simulink model "sm_motor_grader_LiftAssembly"  (R2026a)
settings: Solver=daessc  StopTime=stopTime  AbsTol=1e-3  EnableMultiTasking=on
PostLoadFcn:
  | set_param([bdroot '/Inputs'],'test_source','Data')
  | set_param([bdroot '/Blade'],'popup_actuator_model','Position');
  | set_param([bdroot '/Drawbar'],'popup_actuator_model','Position');
  | set_param([bdroot '/LiftAssembly'],'popup_actuator_model','Position');
  | set_param([bdroot '/Actuation'],'popup_actuator_model','Position');
  | 
  | set_param([bdroot '/Actuation'],'popup_actuator_model_lift','Position');
  | set_param([bdroot '/LiftAssembly'],'popup_actuator_model_lift','Position');
  | 
  | set_param([bdroot '/Blade'],'popup_blade_ground_contact','None')
  | [activeTestCmds,motGradParams,stopTime] = sm_motor_grader_define_test(motGradParams,'GradingTest');
  | set_param(bdroot,'EnablePacing','off')
InitFcn:
  | sm_motor_grader_config_initLinkBarHole([bdroot '/LiftAssembly'],motGradParams)
undefined symbols (not defined in the file): motGradParams, X, Y, Z
libraries: sm_motor_grader_lib x23, sm_lib x5, nesl_utility x1, sm_vehicle_utilities_lib x1
Description:
  | Copyright 2025-2026 The MathWorks, Inc.
settings Model: Creator=smiller  LastModifiedBy=smiller
settings DataIOCC: SignalLoggingName=logsout_sm_motor_grader_LiftAssembly
settings DebuggingCC: SubsystemReferenceDiagnosticForUnitTest=warning
settings SimscapeCC: SimscapeNominalValues="[{\"value\":\"1\",\"unit\":\"A\"},{\"value\":\"1\",\"unit\":\"bar\"},{\"value\":\"1\",\"unit\":\"cm^2\"},{\"value\":\"1\",\"unit\":\"cm^3/s\"},{\"value\":\"1\",\"unit\":\"kJ/kg\"},{\"value\":\"1\",\"unit\":\"kW\"},{\"value\":\"1\",\"unit\":\"l\"},{\"value\":\"1\",\"unit\":\"N\"},{\"value\":\"1\",\"unit\":\"N*m\"},{\"value\":\"1\",\"unit\":\"V\"}]"  SimscapeLogSimulationStatistics=on  SimscapeLogName=simlog_sm_motor_grader_LiftAssembly
settings DiagnosticsConfigSet: SimMechanicsConflictingReferenceFrames=none
settings ExplorerConfigSet: InternalSimMechanicsExplorerSettings="<ExplorerConfiguration><canonicalview>default</canonicalview><AnimationSetting><BasePlaybackSpeed>1.0</BasePlaybackSpeed><PlaybackSpeedFactor>2.0</PlaybackSpeedFactor></AnimationSetting><TilePanel><TileInfo><Tiles Columns=\"2\" Count=\"3\" Rows=\"2\"><Column Weight=\"0.4582\"/><Column Weight=\"0.5418\"/><Row Weight=\"0.5\"/><Row Weight=\"0.5\"/><Tile Height=\"1\" Width=\"1\" X=\"0\" Y=\"0\"/><Tile Height=\"1\" Width=\"1\" X=\"0\" Y=\"1\"/><Tile Height=\"2\" Width=\"1\" X=\"1\" Y=\"0\"/></Tiles></TileInfo><SceneInfo><SceneViewer><BGColor><R>1</R><G>1</G><B>1</B></BGColor><Camera><DoPerspective>off</DoPerspective><Position><X>3.15625000000000044</X><Y>-5.23852944873328152e-32</Y><Z>5.47808148799324002</Z></Position><Center><X>3.15625000000000044</X><Y>-5.23852944873328152e-32</Y><Z>1.95604989013671826</Z></Center><Up><X>0</X><Y>1</Y><Z>0</Z></Up><ViewLimDist>1</ViewLimDist><YLim>2.57500000000000018</YLim><XLim>5.23247330960854118</XLim></Camera></SceneViewer><SceneViewer><BGColor><R>1</R><G>1</G><B>1</B></BGColor><Camera><DoPerspective>off</DoPerspective><Position><X>5.88186405066405449</X><Y>-3.15203884044619187</Y><Z>2.76526245490202038</Z></Position><Center><X>2.73782296717336138</X><Y>0.286756094621752888</Y><Z>1.70087354642860866</Z></Center><Up><X>-0.15027157805512012</X><Y>0.164359538497787616</Y><Z>0.974886862632591944</Z></Up><ViewLimDist>1</ViewLimDist><YLim>2.68459397792816157</YLim><XLim>5.45517139287181596</XLim></Camera></SceneViewer><SceneViewer><BGColor><R>1</R><G>1</G><B>1</B></BGColor><Camera><DoPerspective>off</DoPerspective><Position><X>-0.999784568848335997</X><Y>-2.06162958506149385</Y><Z>2.58851070440858155</Z></Position><Center><X>3.20360113123811852</X><Y>0.528944126100773016</Y><Z>1.25033386358515286</Z></Center><Up><X>0.230558082822453991</X><Y>0.124417230540786017</Y><Z>0.965071667385275167</Z></Up><ViewLimDist>1</ViewLimDist><YLim>3.04628555505233445</YLim><XLim>3.60646065711975128</XLim></Camera></SceneViewer></SceneInfo></TilePanel><MechEditorPanel><Cameras><Camera><Id>Camera1</Id><Value><Name>Track FixO FR</Name><NativeCamera><PositionTrackingFeature>Motor_Grader.Vehicle.Camera_Frames.Frame_FixO_FR.R</PositionTrackingFeature><CenterTrackingFeature>Motor_Grader.Vehicle.Camera_Frames.Frame_FixO_FR.R</CenterTrackingFeature><UpVectorTrackingFeature>Motor_Grader.Vehicle.Camera_Frames.Frame_FixO_FR.R</UpVectorTrackingFeature><CenterTrackingOrigin>off</CenterTrackingOrigin><CenterTrackingDirection>+X</CenterTrackingDirection><UpVectorTrackingDirection>+Z</UpVectorTrackingDirection></NativeCamera></Value></Camera><Camera><Id>Camera2</Id><Value><Name>Track FixO Right</Name><NativeCamera><PositionTrackingFeature>Motor_Grader.Vehicle.Camera_Frames.Frame_FixO_Right.R</PositionTrackingFeature><CenterTrackingFeature>Motor_Grader.Vehicle.Camera_Frames.Frame_FixO_Right.R</CenterTrackingFeature><UpVectorTrackingFeature>Motor_Grader.Vehicle.Camera_Frames.Frame_FixO_Right.R</UpVectorTrackingFeature><CenterTrackingOrigin>off</CenterTrackingOrigin><CenterTrackingDirection>+X</CenterTrackingDirection><UpVectorTrackingDirection>+Z</UpVectorTrackingDirection></NativeCamera></Value></Camera><Camera><Id>Camera3</Id><Value><Name>Track FixO RR</Name><NativeCamera><PositionTrackingFeature>Motor_Grader.Vehicle.Camera_Frames.Frame_FixO_RR.R</PositionTrackingFeature><CenterTrackingFeature>Motor_Grader.Vehicle.Camera_Frames.Frame_FixO_RR.R</CenterTrackingFeature><UpVectorTrackingFeature>Motor_Grader.Vehicle.Camera_Frames.Frame_FixO_RR.R</UpVectorTrackingFeature><CenterTrackingOrigin>off</CenterTrackingOrigin><CenterTrackingDirection>+X</CenterTrackingDirection><UpVectorTrackingDirection>+Z</UpVectorTrackingDirection></NativeCamera></Value></Camera><Camera><Id>Camera4</Id><Value><Name>Track FixO RL</Name><NativeCamera><PositionTrackingFeature>Motor_Grader.Vehicle.Camera_Frames.Frame_FixO_RL.R</PositionTrackingFeature><CenterTrackingFeature>Motor_Grader.Vehicle.Camera_Frames.Frame_FixO_RL.R</CenterTrackingFeature><UpVectorTrackingFeature>Motor_Grader.Vehicle.Camera_Frames.Frame_FixO_RL.R</UpVectorTrackingFeature><CenterTrackingOrigin>off</CenterTrackingOrigin><CenterTrackingDirection>+X</CenterTrackingDirection><UpVectorTrackingDirection>+Z</UpVectorTrackingDirection></NativeCamera></Value></Camera><Camera><Id>Camera5</Id><Value><Name>Track FixO Left</Name><NativeCamera><PositionTrackingFeature>Motor_Grader.Vehicle.Camera_Frames.Frame_FixO_Left.R</PositionTrackingFeature><CenterTrackingFeature>Motor_Grader.Vehicle.Camera_Frames.Frame_FixO_Left.R</CenterTrackingFeature><UpVectorTrackingFeature>Motor_Grader.Vehicle.Camera_Frames.Frame_FixO_Left.R</UpVectorTrackingFeature><CenterTrackingOrigin>off</CenterTrackingOrigin><CenterTrackingDirection>+X</CenterTrackingDirection><UpVectorTrackingDirection>+Z</UpVectorTrackingDirection></NativeCamera></Value></Camera><Camera><Id>Camera6</Id><Value><Name>Track FixO FL</Name><NativeCamera><PositionTrackingFeature>Motor_Grader.Vehicle.Camera_Frames.Frame_FixO_FL.R</PositionTrackingFeature><CenterTrackingFeature>Motor_Grader.Vehicle.Camera_Frames.Frame_FixO_FL.R</CenterTrackingFeature><UpVectorTrackingFeature>Motor_Grader.Vehicle.Camera_Frames.Frame_FixO_FL.R</UpVectorTrackingFeature><CenterTrackingOrigin>off</CenterTrackingOrigin><CenterTrackingDirection>+X</CenterTrackingDirection><UpVectorTrackingDirection>+Z</UpVectorTrackingDirection></NativeCamera></Value></Camera><Camera><Id>Camera7</Id><Value><Name>Track FixO Top</Name><NativeCamera><PositionTrackingFeature>Motor_Grader.Vehicle.Camera_Frames.Frame_FixO_Top.R</PositionTrackingFeature><CenterTrackingFeature>Motor_Grader.Vehicle.Camera_Frames.Frame_FixO_Top.R</CenterTrackingFeature><UpVectorTrackingFeature>Motor_Grader.Vehicle.Camera_Frames.Frame_FixO_Top.R</UpVectorTrackingFeature><CenterTrackingOrigin>off</CenterTrackingOrigin><CenterTrackingDirection>+X</CenterTrackingDirection><UpVectorTrackingDirection>+Z</UpVectorTrackingDirection></NativeCamera></Value></Camera><Camera><Id>Camera8</Id><Value><Name>Track FixO Front</Name><NativeCamera><PositionTrackingFeature>Motor_Grader.Vehicle.Camera_Frames.Frame_FixO_Front.R</PositionTrackingFeature><CenterTrackingFeature>Motor_Grader.Vehicle.Camera_Frames.Frame_FixO_Front.R</CenterTrackingFeature><UpVectorTrackingFeature>Motor_Grader.Vehicle.Camera_Frames.Frame_FixO_Front.R</UpVectorTrackingFeature><CenterTrackingOrigin>off</CenterTrackingOrigin><CenterTrackingDirection>+X</CenterTrackingDirection><UpVectorTrackingDirection>+Z</UpVectorTrackingDirection></NativeCamera></Value></Camera><Camera><Id>Camera9</Id><Value><Name>Track FixO Rear</Name><NativeCamera><PositionTrackingFeature>Motor_Grader.Vehicle.Camera_Frames.Frame_FixO_Rear.R</PositionTrackingFeature><CenterTrackingFeature>Motor_Grader.Vehicle.Camera_Frames.Frame_FixO_Rear.R</CenterTrackingFeature><UpVectorTrackingFeature>Motor_Grader.Vehicle.Camera_Frames.Frame_FixO_Rear.R</UpVectorTrackingFeature><CenterTrackingOrigin>off</CenterTrackingOrigin><CenterTrackingDirection>+X</CenterTrackingDirection><UpVectorTrackingDirection>+Z</UpVectorTrackingDirection></NativeCamera></Value></Camera><Camera><Id>Camera10</Id><Value><Name>Track FR</Name><NativeCamera><PositionTrackingFeature>Motor_Grader.Vehicle.Camera_Frames.Frame_FR.R</PositionTrackingFeature><CenterTrackingFeature>Motor_Grader.Vehicle.Camera_Frames.Frame_FR.R</CenterTrackingFeature><UpVectorTrackingFeature>Motor_Grader.Vehicle.Camera_Frames.Frame_FR.R</UpVectorTrackingFeature><CenterTrackingOrigin>off</CenterTrackingOrigin><CenterTrackingDirection>+X</CenterTrackingDirection><UpVectorTrackingDirection>+Z</UpVectorTrackingDirection></NativeCamera></Value></Camera><Camera><Id>Camera11</Id><Value><Name>Track Right</Name><NativeCamera><PositionTrackingFeature>Motor_Grader.Vehicle.Camera_Frames.Frame_Right.R</PositionTrackingFeature><CenterTrackingFeature>Motor_Grader.Vehicle.Camera_Frames.Frame_Right.R</CenterTrackingFeature><UpVectorTrackingFeature>Motor_Grader.Vehicle.Camera_Frames.Frame_Right.R</UpVectorTrackingFeature><CenterTrackingOrigin>off</CenterTrackingOrigin><CenterTrackingDirection>+X</CenterTrackingDirection><UpVectorTrackingDirection>+Z</UpVectorTrackingDirection></NativeCamera></Value></Camera><Camera><Id>Camera12</Id><Value><Name>Track RR</Name><NativeCamera><PositionTrackingFeature>Motor_Grader.Vehicle.Camera_Frames.Frame_RR.R</PositionTrackingFeature><CenterTrackingFeature>Motor_Grader.Vehicle.Camera_Frames.Frame_RR.R</CenterTrackingFeature><UpVectorTrackingFeature>Motor_Grader.Vehicle.Camera_Frames.Frame_RR.R</UpVectorTrackingFeature><CenterTrackingOrigin>off</CenterTrackingOrigin><CenterTrackingDirection>+X</CenterTrackingDirection><UpVectorTrackingDirection>+Z</UpVectorTrackingDirection></NativeCamera></Value></Camera><Camera><Id>Camera13</Id><Value><Name>Track RL</Name><NativeCamera><PositionTrackingFeature>Motor_Grader.Vehicle.Camera_Frames.Frame_RL.R</PositionTrackingFeature><CenterTrackingFeature>Motor_Grader.Vehicle.Camera_Frames.Frame_RL.R</CenterTrackingFeature><UpVectorTrackingFeature>Motor_Grader.Vehicle.Camera_Frames.Frame_RL.R</UpVectorTrackingFeature><CenterTrackingOrigin>off</CenterTrackingOrigin><CenterTrackingDirection>+X</CenterTrackingDirection><UpVectorTrackingDirection>+Z</UpVectorTrackingDirection></NativeCamera></Value></Camera><Camera><Id>Camera14</Id><Value><Name>Track Left</Name><NativeCamera><PositionTrackingFeature>Motor_Grader.Vehicle.Camera_Frames.Frame_Left.R</PositionTrackingFeature><CenterTrackingFeature>Motor_Grader.Vehicle.Camera_Frames.Frame_Left.R</CenterTrackingFeature><UpVectorTrackingFeature>Motor_Grader.Vehicle.Camera_Frames.Frame_Left.R</UpVectorTrackingFeature><CenterTrackingOrigin>off</CenterTrackingOrigin><CenterTrackingDirection>+X</CenterTrackingDirection><UpVectorTrackingDirection>+Z</UpVectorTrackingDirection></NativeCamera></Value></Camera><Camera><Id>Camera15</Id><Value><Name>Track FL</Name><NativeCamera><PositionTrackingFeature>Motor_Grader.Vehicle.Camera_Frames.Frame_FL.R</PositionTrackingFeature><CenterTrackingFeature>Motor_Grader.Vehicle.Camera_Frames.Frame_FL.R</CenterTrackingFeature><UpVectorTrackingFeature>Motor_Grader.Vehicle.Camera_Frames.Frame_FL.R</UpVectorTrackingFeature><CenterTrackingOrigin>off</CenterTrackingOrigin><CenterTrackingDirection>+X</CenterTrackingDirection><UpVectorTrackingDirection>+Z</UpVectorTrackingDirection></NativeCamera></Value></Camera><Camera><Id>Camera16</Id><Value><Name>Track Top</Name><NativeCamera><PositionTrackingFeature>Motor_Grader.Vehicle.Camera_Frames.Frame_Top.R</PositionTrackingFeature><CenterTrackingFeature>Motor_Grader.Vehicle.Camera_Frames.Frame_Top.R</CenterTrackingFeature><UpVectorTrackingFeature>Motor_Grader.Vehicle.Camera_Frames.Frame_Top.R</UpVectorTrackingFeature><CenterTrackingOrigin>off</CenterTrackingOrigin><CenterTrackingDirection>+X</CenterTrackingDirection><UpVectorTrackingDirection>+Z</UpVectorTrackingDirection></NativeCamera></Value></Camera><Camera><Id>Camera17</Id><Value><Name>Track Front</Name><NativeCamera><PositionTrackingFeature>Motor_Grader.Vehicle.Camera_Frames.Frame_Front.R</PositionTrackingFeature><CenterTrackingFeature>Motor_Grader.Vehicle.Camera_Frames.Frame_Front.R</CenterTrackingFeature><UpVectorTrackingFeature>Motor_Grader.Vehicle.Camera_Frames.Frame_Front.R</UpVectorTrackingFeature><CenterTrackingOrigin>off</CenterTrackingOrigin><CenterTrackingDirection>+X</CenterTrackingDirection><UpVectorTrackingDirection>+Z</UpVectorTrackingDirection></NativeCamera></Value></Camera><Camera><Id>Camera18</Id><Value><Name>Track Rear</Name><NativeCamera><PositionTrackingFeature>Motor_Grader.Vehicle.Camera_Frames.Frame_Rear.R</PositionTrackingFeature><CenterTrackingFeature>Motor_Grader.Vehicle.Camera_Frames.Frame_Rear.R</CenterTrackingFeature><UpVectorTrackingFeature>Motor_Grader.Vehicle.Camera_Frames.Frame_Rear.R</UpVectorTrackingFeature><CenterTrackingOrigin>off</CenterTrackingOrigin><CenterTrackingDirection>+X</CenterTrackingDirection><UpVectorTrackingDirection>+Z</UpVectorTrackingDirection></NativeCamera></Value></Camera><Camera><Id>Camera19</Id><Value><Name>Track Blade Front</Name><NativeCamera><PositionTrackingFeature>Motor_Grader.Vehicle.Camera_Frames.Frame_SuspF.R</PositionTrackingFeature><CenterTrackingFeature>Motor_Grader.Vehicle.Camera_Frames.Frame_SuspF.R</CenterTrackingFeature><UpVectorTrackingFeature>Motor_Grader.Vehicle.Camera_Frames.Frame_SuspF.R</UpVectorTrackingFeature><CenterTrackingOrigin>off</CenterTrackingOrigin><CenterTrackingDirection>+X</CenterTrackingDirection><UpVectorTrackingDirection>+Z</UpVectorTrackingDirection></NativeCamera></Value></Camera><Camera><Id>Camera20</Id><Value><Name>Track Blade Rear</Name><NativeCamera><PositionTrackingFeature>Motor_Grader.Vehicle.Camera_Frames.Frame_SuspR.R</PositionTrackingFeature><CenterTrackingFeature>Motor_Grader.Vehicle.Camera_Frames.Frame_SuspR.R</CenterTrackingFeature><UpVectorTrackingFeature>Motor_Grader.Vehicle.Camera_Frames.Frame_SuspR.R</UpVectorTrackingFeature><CenterTrackingOrigin>off</CenterTrackingOrigin><CenterTrackingDirection>+X</CenterTrackingDirection><UpVectorTrackingDirection>+Z</UpVectorTrackingDirection></NativeCamera></Value></Camera><Camera><Id>Camera21</Id><Value><Name>Track Wheel FR</Name><NativeCamera><PositionTrackingFeature>Motor_Grader.Vehicle.Camera_Frames.Frame_Wheel_FR.R</PositionTrackingFeature><CenterTrackingFeature>Motor_Grader.Vehicle.Camera_Frames.Frame_Wheel_FR.R</CenterTrackingFeature><UpVectorTrackingFeature>Motor_Grader.Vehicle.Camera_Frames.Frame_Wheel_FR.R</UpVectorTrackingFeature><CenterTrackingOrigin>off</CenterTrackingOrigin><CenterTrackingDirection>+X</CenterTrackingDirection><UpVectorTrackingDirection>+Z</UpVectorTrackingDirection></NativeCamera></Value></Camera><Camera><Id>Camera22</Id><Value><Name>Track Blade Right</Name><NativeCamera><PositionTrackingFeature>Motor_Grader.Vehicle.Camera_Frames.Frame_Wheel_RR.R</PositionTrackingFeature><CenterTrackingFeature>Motor_Grader.Vehicle.Camera_Frames.Frame_Wheel_RR.R</CenterTrackingFeature><UpVectorTrackingFeature>Motor_Grader.Vehicle.Camera_Frames.Frame_Wheel_RR.R</UpVectorTrackingFeature><CenterTrackingOrigin>off</CenterTrackingOrigin><CenterTrackingDirection>+X</CenterTrackingDirection><UpVectorTrackingDirection>+Z</UpVectorTrackingDirection></NativeCamera></Value></Camera><Camera><Id>Camera23</Id><Value><Name>Track Blade Left</Name><NativeCamera><PositionTrackingFeature>Motor_Grader.Vehicle.Camera_Frames.Frame_Wheel_RL.R</PositionTrackingFeature><CenterTrackingFeature>Motor_Grader.Vehicle.Camera_Frames.Frame_Wheel_RL.R</CenterTrackingFeature><UpVectorTrackingFeature>Motor_Grader.Vehicle.Camera_Frames.Frame_Wheel_RL.R</UpVectorTrackingFeature><CenterTrackingOrigin>off</CenterTrackingOrigin><CenterTrackingDirection>+X</CenterTrackingDirection><UpVectorTrackingDirection>+Z</UpVectorTrackingDirection></NativeCamera></Value></Camera><Camera><Id>Camera24</Id><Value><Name>Track Wheel FL</Name><NativeCamera><PositionTrackingFeature>Motor_Grader.Vehicle.Camera_Frames.Frame_Wheel_FL.R</PositionTrackingFeature><CenterTrackingFeature>Motor_Grader.Vehicle.Camera_Frames.Frame_Wheel_FL.R</CenterTrackingFeature><UpVectorTrackingFeature>Motor_Grader.Vehicle.Camera_Frames.Frame_Wheel_FL.R</UpVectorTrackingFeature><CenterTrackingOrigin>off</CenterTrackingOrigin><CenterTrackingDirection>+X</CenterTrackingDirection><UpVectorTrackingDirection>+Z</UpVectorTrackingDirection></NativeCamera></Value></Camera><Camera><Id>Camera25</Id><Value><Name>View Seat</Name><NativeCamera><PositionTrackingFeature>Motor_Grader.Vehicle.Camera_Frames.Frame_View_Seat_FL.R</PositionTrackingFeature><CenterTrackingFeature>Motor_Grader.Vehicle.Camera_Frames.Frame_View_Seat_FL.R</CenterTrackingFeature><UpVectorTrackingFeature>Motor_Grader.Vehicle.Camera_Frames.Frame_View_Seat_FL.R</UpVectorTrackingFeature><CenterTrackingOrigin>off</CenterTrackingOrigin><CenterTrackingDirection>+X</CenterTrackingDirection><UpVectorTrackingDirection>+Z</UpVectorTrackingDirection></NativeCamera></Value></Camera><Camera><Id>Camera26</Id><Value><Name>View Seat FR</Name><NativeCamera><PositionTrackingFeature>Motor_Grader.Vehicle.Camera_Frames.Frame_View_Seat_FR.R</PositionTrackingFeature><CenterTrackingFeature>Motor_Grader.Vehicle.Camera_Frames.Frame_View_Seat_FR.R</CenterTrackingFeature><UpVectorTrackingFeature>Motor_Grader.Vehicle.Camera_Frames.Frame_View_Seat_FR.R</UpVectorTrackingFeature><CenterTrackingOrigin>off</CenterTrackingOrigin><CenterTrackingDirection>+X</CenterTrackingDirection><UpVectorTrackingDirection>+Z</UpVectorTrackingDirection></NativeCamera></Value></Camera><Camera><Id>Camera27</Id><Value><Name>View Susp FR</Name><NativeCamera><PositionTrackingFeature>Motor_Grader.Vehicle.Camera_Frames.Frame_View_Susp_FR.R</PositionTrackingFeature><CenterTrackingFeature>Motor_Grader.Vehicle.Camera_Frames.Frame_View_Susp_FR.R</CenterTrackingFeature><UpVectorTrackingFeature>Motor_Grader.Vehicle.Camera_Frames.Frame_View_Susp_FR.R</UpVectorTrackingFeature><CenterTrackingOrigin>off</CenterTrackingOrigin><CenterTrackingDirection>+X</CenterTrackingDirection><UpVectorTrackingDirection>+Z</UpVectorTrackingDirection></NativeCamera></Value></Camera><Camera><Id>Camera28</Id><Value><Name>View SaddleR</Name><NativeCamera><PositionTrackingFeature>Motor_Grader.Vehicle.Camera_Frames.Frame_View_Susp_RR.R</PositionTrackingFeature><CenterTrackingFeature>Motor_Grader.Vehicle.Camera_Frames.Frame_View_Susp_RR.R</CenterTrackingFeature><UpVectorTrackingFeature>Motor_Grader.Vehicle.Camera_Frames.Frame_View_Susp_RR.R</UpVectorTrackingFeature><CenterTrackingOrigin>off</CenterTrackingOrigin><CenterTrackingDirection>+X</CenterTrackingDirection><UpVectorTrackingDirection>+Z</UpVectorTrackingDirection></NativeCamera></Value></Camera><Camera><Id>Camera29</Id><Value><Name>View SaddleL</Name><NativeCamera><PositionTrackingFeature>Motor_Grader.Vehicle.Camera_Frames.Frame_View_Susp_RL.R</PositionTrackingFeature><CenterTrackingFeature>Motor_Grader.Vehicle.Camera_Frames.Frame_View_Susp_RL.R</CenterTrackingFeature><UpVectorTrackingFeature>Motor_Grader.Vehicle.Camera_Frames.Frame_View_Susp_RL.R</UpVectorTrackingFeature><CenterTrackingOrigin>off</CenterTrackingOrigin><CenterTrackingDirection>+X</CenterTrackingDirection><UpVectorTrackingDirection>+Z</UpVectorTrackingDirection></NativeCamera></Value></Camera><Camera><Id>Camera30</Id><Value><Name>View Susp FL</Name><NativeCamera><PositionTrackingFeature>Motor_Grader.Vehicle.Camera_Frames.Frame_View_Susp_FL.R</PositionTrackingFeature><CenterTrackingFeature>Motor_Grader.Vehicle.Camera_Frames.Frame_View_Susp_FL.R</CenterTrackingFeature><UpVectorTrackingFeature>Motor_Grader.Vehicle.Camera_Frames.Frame_View_Susp_FL.R</UpVectorTrackingFeature><CenterTrackingOrigin>off</CenterTrackingOrigin><CenterTrackingDirection>+X</CenterTrackingDirection><UpVectorTrackingDirection>+Z</UpVectorTrackingDirection></NativeCamera></Value></Camera><Camera><Id>Camera31</Id><Value><Name>Dolly Camera</Name><NativeCamera><PositionTrackingFeature>Motor_Grader.Vehicle.Camera_Frames.Frame_Dolly.R</PositionTrackingFeature><CenterTrackingFeature>Motor_Grader.Vehicle.Camera_Frames.Frame_Dolly.R</CenterTrackingFeature><UpVectorTrackingFeature>Motor_Grader.Vehicle.Camera_Frames.Frame_Dolly.R</UpVectorTrackingFeature><CenterTrackingOrigin>off</CenterTrackingOrigin><CenterTrackingDirection>+X</CenterTrackingDirection><UpVectorTrackingDirection>+Z</UpVectorTrackingDirection></NativeCamera></Value></Camera><Camera><Id>Camera32</Id><Value><Name>Track Dolly Camera</Name><NativeCamera><PositionTrackingFeature>Motor_Grader.Vehicle.Camera_Frames.Frame_Dolly.R</PositionTrackingFeature><CenterTrackingFeature>Motor_Grader.Vehicle.Camera_Frames.Transform_Camera_Ref.F</CenterTrackingFeature><UpVectorTrackingFeature>Motor_Grader.Vehicle.Camera_Frames.World_Frame.W</UpVectorTrackingFeature><CenterTrackingOrigin>on</CenterTrackingOrigin><UpVectorTrackingDirection>+Z</UpVectorTrackingDirection></NativeCamera></Value></Camera></Cameras><GfxPanelCameraMap/><VideoCreator><PlaybackSpeedRatio>1.0</PlaybackSpeedRatio><FrameRate>30</FrameRate><VideoFormat>MPEG-4</VideoFormat><FrameSize>[800 450]</FrameSize></VideoCreator></MechEditorPanel></ExplorerConfiguration>"

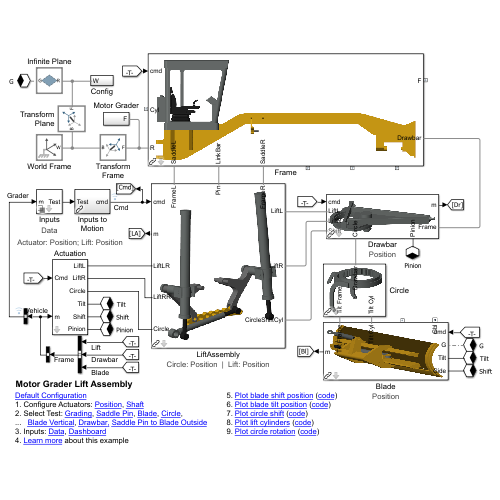
[thumbnail: Simulink's stored preview of the top-level diagram]
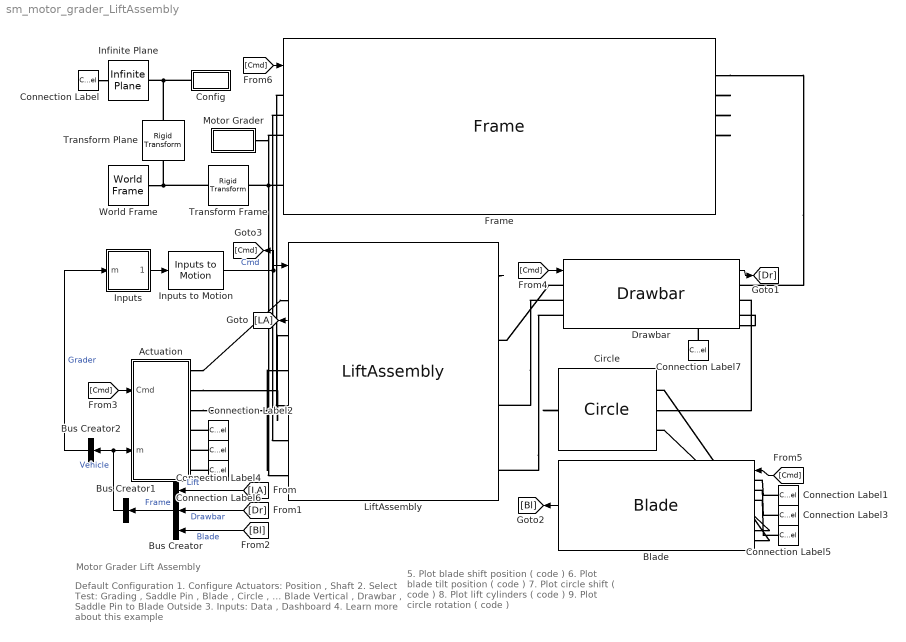
== system sm_motor_grader_LiftAssembly ==
  note: Motor Grader Lift Assembly
  note: Default Configuration
      | 1. Configure Actuators: Position , Shaft
      | 2. Select Test: Grading , Saddle Pin , Blade , Circle ,
      | ... Blade Vertical , Drawbar , Saddle Pin to Blade Outside
      | 3. Inputs: Data , Dashboard
      | 4. Learn more about this example
  note: 5. Plot blade shift position ( code )
      | 6. Plot blade tilt position ( code )
      | 7. Plot circle shift ( code )
      | 8. Plot lift cylinders ( code )
      | 9. Plot circle rotation ( code )
  Actuation : Subsystem  VariantControl=Actuation  mask{popup_actuator_model=Position, popup_actuator_model_lift=Position}
      mask prompts: popup_actuator_model "Actuation Mode"; popup_actuator_model_lift "Actuation Mode Lift"
      mask init:
      | bh = gcb;
      | modestr = get_param(bh,'popup_actuator_model');
      | set_param([bh '/Actuator Circle'],'LabelModeActiveChoice',modestr)
      | set_param([bh '/Actuator Tilt'],'LabelModeActiveChoice',modestr)
      | set_param([bh '/Actuator Shift'],'LabelModeActiveChoice',modestr)
      | set_param([bh '/Actuator Pinion'],'LabelModeActiveChoice',modestr)
      | 
      | liftmodestr = get_param(bh,'popup_actuator_model_lift');
      | set_param([bh '/Actuator LiftL'],'LabelModeActiveChoice',liftmodestr)
      | set_param([bh '/Actuator LiftR'],'LabelModeActiveChoice',liftmodestr)
      settings: AttributesFormatString=Actuator: %<popup_actuator_model>; Lift: %<popup_actuator_model_lift>
      mask TypeOptions popup_actuator_model: Position | Shaft
      mask TypeOptions popup_actuator_model_lift: Position | Shaft
  Blade : sm_motor_grader_lib/Blade  popup_actuator_model=Position  popup_blade_ground_contact=None
      settings: AttributesFormatString=%<popup_actuator_model>
  Bus Creator : BusCreator  Inputs=3
  Bus Creator1 : BusCreator  Inputs=1
  Bus Creator2 : BusCreator  Inputs=1
  Circle : sm_motor_grader_lib/Circle
  Config : Subsystem
  Connection Label : ConnectionLabel  Label=G
  Connection Label1 : ConnectionLabel  Label=G
  Connection Label2 : ConnectionLabel  Label=Tilt
  Connection Label3 : ConnectionLabel  Label=Tilt
  Connection Label4 : ConnectionLabel  Label=Shift
  Connection Label5 : ConnectionLabel  Label=Shift
  Connection Label6 : ConnectionLabel  Label=Pinion
  Connection Label7 : ConnectionLabel  Label=Pinion
  Drawbar : sm_motor_grader_lib/Drawbar  popup_actuator_model=Position
      settings: AttributesFormatString=%<popup_actuator_model>
  Frame : sm_motor_grader_lib/Frame
  Infinite Plane : sm_lib/Curves and Surfaces/Infinite Plane  GraphicType=Rectangle  GraphicPlaneWidth=6  GraphicPlaneWidthUnits=m  GraphicPlaneHeight=5  GraphicPlaneHeightUnits=m  GraphicVisPropType=SimpleVisualProperties  GraphicDiffuseColor=[0.5 0.5 0.5]  GraphicOpacity=0.5  GraphicSpecularColor=[0.5 0.5 0.5 1.0]  GraphicAmbientColor=[0.15 0.15 0.15 1.0]  GraphicEmissiveColor=[0.0 0.0 0.0 1.0]  GraphicShininess=75
  Inputs : Subsystem  Variant=on  VariantControlMode=label  VariantControl=Inputs  LabelModeActiveChoice=Data  mask{test_source=Data}
      mask prompts: test_source "Test Source"
      mask init:
      | bh = gcb;
      | data_source = get_param(bh,'test_source');
      | set_param(bh,'LabelModeActiveChoice',data_source)
      settings: AttributesFormatString=%<LabelModeActiveChoice>
      mask TypeOptions test_source: Data | Dashboard
      mask Display: disp(' ')
  Inputs to Motion : sm_motor_grader_lib/Inputs to Motion  SystemSampleTime=-1  VariantActivationTime=update diagram  EmptyChoice=off  PassThrough=off  PassThroughVariantControl=(default)  EmptyChoiceVariantControl=(default)  AllowFlexibleInterface=on  Latency=0  AutoFrameSizeCalculation=off
  LiftAssembly : sm_motor_grader_lib/LiftAssembly  popup_actuator_model=Position  popup_actuator_model_lift=Position  popup_initial_hole=Center
      settings: AttributesFormatString="Circle: %<popup_actuator_model>  |  Lift: %<popup_actuator_model_lift>"
  Motor Grader : Subsystem
  Transform Frame : sm_lib/Frames and Transforms/Rigid Transform  RotationMethod=None  FollAlignAxisA=+X  BaseAlignAxisA=+Y  FollAlignAxisB=+Y  BaseAlignAxisB=+Z  RotationStandardAxis=+Z  RotationAngle=0.0  RotationAngleUnits=deg  RotationArbitraryAxis=[0 0 1]  RotationSequenceAxes=FollowerAxes  RotationSequence=XYX  RotationSequenceAngles=[0 0 0]  RotationSequenceAnglesUnits=deg  RotationMatrix=[1 0 0; 0 1 0; 0 0 1]  Quaternion=[1 0 0 0]  TranslationMethod=StandardAxis  TranslationCartesianOffset=[0 0 0]  TranslationCartesianOffsetUnits=m  TranslationStandardAxis=+Z  TranslationStandardOffset=1.0871  TranslationStandardOffsetUnits=m  TranslationROffset=0  TranslationROffsetUnits=m  TranslationThetaOffset=0  TranslationThetaOffsetUnits=deg  TranslationZOffset=0  TranslationZOffsetUnits=m
  Transform Plane : sm_lib/Frames and Transforms/Rigid Transform  RotationMethod=None  FollAlignAxisA=+X  BaseAlignAxisA=+Y  FollAlignAxisB=+Y  BaseAlignAxisB=+Z  RotationStandardAxis=+Z  RotationAngle=0  RotationAngleUnits=deg  RotationArbitraryAxis=[0 0 1]  RotationSequenceAxes=FollowerAxes  RotationSequence=XYX  RotationSequenceAngles=[0 0 0]  RotationSequenceAnglesUnits=deg  RotationMatrix=[1 0 0;0 1 0;0 0 1]  Quaternion=[1 0 0 0]  TranslationMethod=StandardAxis  TranslationCartesianOffset=[0 0 0]  TranslationCartesianOffsetUnits=m  TranslationStandardAxis=+X  TranslationStandardOffset=3  TranslationStandardOffsetUnits=m  TranslationROffset=0  TranslationROffsetUnits=m  TranslationThetaOffset=0  TranslationThetaOffsetUnits=deg  TranslationZOffset=0  TranslationZOffsetUnits=m
  World Frame : sm_lib/Frames and Transforms/World Frame
  wires:
  Inputs to Motion/1 -> LiftAssembly/1, [Cmd]  "Cmd"
  LiftAssembly/1 -> [LA]
  Drawbar/1 -> [Dr]
  [LA] -> Bus Creator/1  "Lift"
  [Dr] -> Bus Creator/2  "Drawbar"
  Bus Creator/1 -> Bus Creator1/1  "Frame"
  Blade/1 -> [Bl]
  [Bl] -> Bus Creator/3  "Blade"
  Bus Creator1/1 -> Bus Creator2/1, Actuation/2(m)  "Vehicle"
  [Cmd] -> Actuation/1(Cmd)
  [Cmd] -> Blade/1
  [Cmd] -> Frame/1
  [Cmd] -> Drawbar/1
  Inputs/1(Test) -> Inputs to Motion/1
  Bus Creator2/1 -> Inputs/1(m)  "Grader"
  connections:
  Frame/LConn2 -- Motor Grader/RConn1 -- Transform Frame/RConn1
  Frame/RConn3 -- LiftAssembly/LConn4
  Frame/RConn4 -- LiftAssembly/LConn5
  Frame/RConn5 -- LiftAssembly/LConn6
  Actuation/RConn1 -- LiftAssembly/LConn1
  Actuation/RConn2 -- LiftAssembly/LConn2
  Actuation/RConn3 -- LiftAssembly/LConn3
  Drawbar/LConn1 -- LiftAssembly/RConn1
  Drawbar/LConn2 -- LiftAssembly/RConn2
  Drawbar/LConn3 -- LiftAssembly/RConn3
  Frame/RConn2 -- Drawbar/RConn1
  Blade/LConn6 -- Circle/RConn2
  Circle/LConn1 -- Drawbar/RConn2
  Blade/LConn7 -- Circle/RConn1
  Connection Label/LConn1 -- Infinite Plane/RConn1
  Connection Label1/LConn1 -- Blade/LConn1
  World Frame/RConn1 -- Transform Frame/LConn1 -- Transform Plane/LConn1
  Connection Label2/LConn1 -- Actuation/RConn4
  Connection Label3/LConn1 -- Blade/LConn2
  Connection Label4/LConn1 -- Actuation/RConn5
  Connection Label5/LConn1 -- Blade/LConn3
  Connection Label6/LConn1 -- Actuation/RConn6
  Connection Label7/LConn1 -- Drawbar/RConn3
  Transform Plane/RConn1 -- Config/LConn1 -- Infinite Plane/LConn1

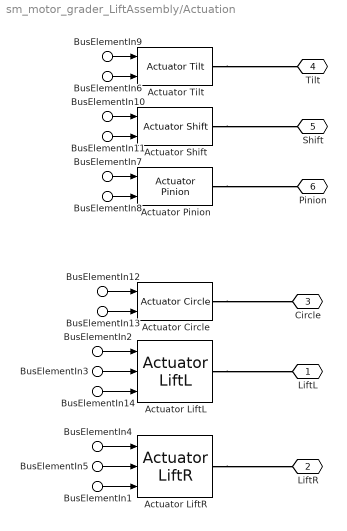
== system sm_motor_grader_LiftAssembly/Actuation ==
  BusElementIn2 : Inport  PortName=Cmd  Element=pLiftL
  BusElementIn4 : Inport  PortName=Cmd  Element=pLiftR
  BusElementIn12 : Inport  PortName=Cmd  Element=pCircleShift
  BusElementIn10 : Inport  PortName=Cmd  Element=pShift
  BusElementIn9 : Inport  PortName=Cmd  Element=pTilt
  BusElementIn7 : Inport  PortName=Cmd  Element=qCircle
  BusElementIn14 : Inport  PortName=Cmd  Element=mLiftL
  BusElementIn1 : Inport  PortName=Cmd  Element=mLiftR
  BusElementIn6 : Inport  Port=2  PortName=m  Element=Frame.Blade.Tilt.p
  BusElementIn11 : Inport  Port=2  PortName=m  Element=Frame.Blade.Shift.p
  BusElementIn3 : Inport  Port=2  PortName=m  Element=Frame.Lift.LiftL.p
  BusElementIn5 : Inport  Port=2  PortName=m  Element=Frame.Lift.LiftR.p
  BusElementIn13 : Inport  Port=2  PortName=m  Element=Frame.Lift.CircleShift.p
  BusElementIn8 : Inport  Port=2  PortName=m  Element=Frame.Drawbar.Circle.q
  Actuator Circle : sm_motor_grader_lib/Actuation/Actuator Circle  SystemSampleTime=-1  VariantControl=Actuator Circle  LabelModeActiveChoice=Position  VariantActivationTime=update diagram  EmptyChoice=off  PassThrough=off  PassThroughVariantControl=(default)  EmptyChoiceVariantControl=(default)  AllowFlexibleInterface=on  Latency=0  AutoFrameSizeCalculation=off
  Actuator LiftL : sm_motor_grader_lib/Actuation/Actuator LiftL  SystemSampleTime=-1  VariantControl=Actuator LiftL  LabelModeActiveChoice=Position  VariantActivationTime=update diagram  EmptyChoice=off  PassThrough=off  PassThroughVariantControl=(default)  EmptyChoiceVariantControl=(default)  AllowFlexibleInterface=on  Latency=0  AutoFrameSizeCalculation=off
  Actuator LiftR : sm_motor_grader_lib/Actuation/Actuator LiftR  SystemSampleTime=-1  VariantControl=Actuator LiftR  LabelModeActiveChoice=Position  VariantActivationTime=update diagram  EmptyChoice=off  PassThrough=off  PassThroughVariantControl=(default)  EmptyChoiceVariantControl=(default)  AllowFlexibleInterface=on  Latency=0  AutoFrameSizeCalculation=off
  Actuator Pinion : sm_motor_grader_lib/Actuation/Actuator Pinion  SystemSampleTime=-1  VariantControl=Actuator Pinion  LabelModeActiveChoice=Position  VariantActivationTime=update diagram  EmptyChoice=off  PassThrough=off  PassThroughVariantControl=(default)  EmptyChoiceVariantControl=(default)  AllowFlexibleInterface=on  Latency=0  AutoFrameSizeCalculation=off
  Actuator Shift : sm_motor_grader_lib/Actuation/Actuator Shift  VariantControl=Actuator Shift  LabelModeActiveChoice=Position
  Actuator Tilt : sm_motor_grader_lib/Actuation/Actuator Tilt  VariantControl=Actuator Tilt  LabelModeActiveChoice=Position
  LiftL : PMIOPort  Side=Right
  LiftR : PMIOPort  Port=2  Side=Right
  Circle : PMIOPort  Port=3  Side=Right
  Tilt : PMIOPort  Port=4  Side=Right
  Shift : PMIOPort  Port=5  Side=Right
  Pinion : PMIOPort  Port=6  Side=Right
  wires:
  BusElementIn12/1 -> Actuator Circle/1
  BusElementIn13/1 -> Actuator Circle/2
  BusElementIn2/1 -> Actuator LiftL/1
  BusElementIn3/1 -> Actuator LiftL/2
  BusElementIn14/1 -> Actuator LiftL/3
  BusElementIn4/1 -> Actuator LiftR/1
  BusElementIn5/1 -> Actuator LiftR/2
  BusElementIn1/1 -> Actuator LiftR/3
  BusElementIn10/1 -> Actuator Shift/1
  BusElementIn6/1 -> Actuator Tilt/2
  BusElementIn11/1 -> Actuator Shift/2
  BusElementIn9/1 -> Actuator Tilt/1
  BusElementIn7/1 -> Actuator Pinion/1
  BusElementIn8/1 -> Actuator Pinion/2
  connections:
  Actuator Circle/RConn1 -- Circle/RConn1
  Actuator LiftL/RConn1 -- LiftL/RConn1
  Actuator LiftR/RConn1 -- LiftR/RConn1
  Actuator Tilt/RConn1 -- Tilt/RConn1
  Actuator Shift/RConn1 -- Shift/RConn1
  Actuator Pinion/RConn1 -- Pinion/RConn1

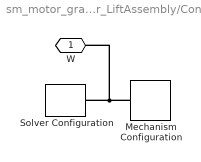
== system sm_motor_grader_LiftAssembly/Config ==
  Mechanism Configuration : sm_lib/Utilities/Mechanism Configuration  UniformGravity=Constant  GravityVector=[0 0 -9.80665]  GravityVectorUnits=m/s^2  LinearizationDelta=0.001  JointModeTransitionNonlinearIterations=2
  Solver Configuration : nesl_utility/Solver Configuration  PhysicalDomain=network_engine_domain  SubClassName=solver  LeftPortType=input  RightPortType=generic  Tones=[]  Harmonics=[]  SimulateNoise=off  Profile=off  UseLocalSampling=off  EnableSwitchedLinearOptims=on  FrequencyDomain=off  UseCCode=off  RelTol=0.001  AbsTol=1e-06  MinStep=1e-09  ToWorkspace=off  RevertToSquareIcSolve=off  NumHomotopyIterations=100  PhasorMode=off  PhasorModeNumHarmonics=1  ConsistencySolver=NEWTON_XTOL_AFTER_FTOL  CanonicalOrdering=UNORDERED  OptimizeIntermediates=UNOPTIMIZED  IndexReductionMethod=DerivativeReplacement  DoDC=off  ResidualTolerance=1e-09  ConsistencyTolSource=GLOBAL  ConsistencyAbsTol=0.001  ConsistencyRelTol=0.001  ConsistencyTolFactor=0.001  UseLocalSolver=off  LocalSolverChoice=NE_BACKWARD_EULER_ADVANCER  ResolveIndetEquations=on  FunctionEvalNumThread=1  LocalSolverSampleTime=0.001  DoFixedCost=off  MaxNonlinIter=3  MaxModeIter=2  ComputeImpulses=off  ImpulseIterations=2  LinearAlgebra=Sparse  LinearAlgebraNumThread=0  EquationFormulation=NE_TIME_EF  DelaysMemoryBudget=1024  AutomaticFiltering=on  FilteringTimeConstant=0.001  PartitionStorageMethod=AS_NEEDED  PartitionMemoryBudget=1024  PartitionMethod=FAST  MultibodyUseLocalSolver=off  MultibodyLocalSolverChoice=ODE1  MultibodyLocalSolverSampleTime=0.001
  W : PMIOPort  Side=Left
  connections:
  Mechanism Configuration/RConn1 -- W/RConn1 -- Solver Configuration/RConn1

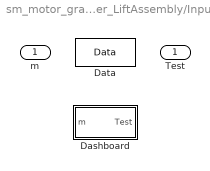
== system sm_motor_grader_LiftAssembly/Inputs ==
  m : Inport
  Dashboard : Subsystem  VariantControl=Dashboard
  Data : sm_motor_grader_lib/Data  SystemSampleTime=-1  VariantControl=Data  VariantActivationTime=update diagram  EmptyChoice=off  PassThrough=off  PassThroughVariantControl=(default)  EmptyChoiceVariantControl=(default)  AllowFlexibleInterface=on  Latency=0  AutoFrameSizeCalculation=off
  Test : Outport

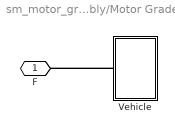
== system sm_motor_grader_LiftAssembly/Motor Grader ==
  Vehicle : Subsystem
  F : PMIOPort  Side=Right
  connections:
  Vehicle/RConn1 -- F/RConn1

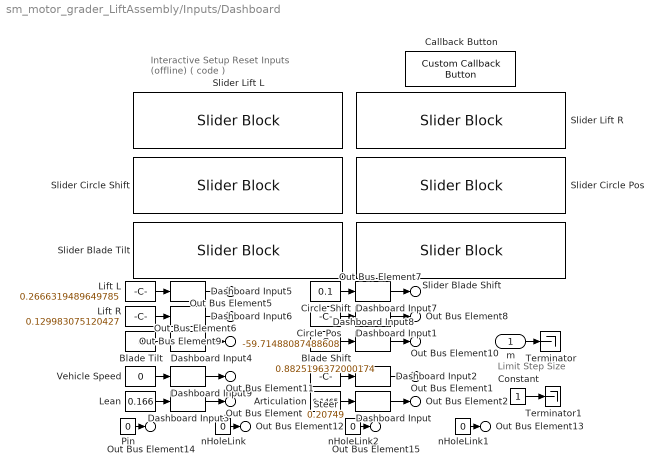
== system sm_motor_grader_LiftAssembly/Inputs/Dashboard ==
  note: Limit Step Size
  note: Interactive Setup
      | Reset Inputs (offline) ( code )
  m : Inport
  Articulation : Constant  Value=0.1465
  Blade Shift : Constant  Value=0.8825196372000174
  Blade Tilt : Constant  Value=0
  Callback Button : CustomCallbackButton  Configuration="{\"components\":[{\"name\":\"BackgroundImageComponent\",\"settings\":{\"image\":{\"size\":[0,0],\"src\":\"default\",\"srcOrientation\":\"Right\"},\"position\":[0,0,1,1]}},{\"name\":\"ButtonStateComponent\",\"settings\":{\"buttonType\":\"momentary\",\"clickFcn\":\"sm_motor_grader_init_dashboard_values(gcs,motGradParams)\",\"onValue\":1,\"position\":[0,0,1,1],\"pressDelay\":\"500\",\"pressFcn\":\"\",\"repeatInterval\":\"0\",\"states\":[{\"horizontalAlignment\":\"center\",\"image\":{\"position\":[0,0,1,1],\"size\":[1,1],\"src\":\"default\",\"srcOrientation\":\"Right\"},\"label\":{\"color\":[0.01176470588,0.01176470588,0.01176470588,1],\"icon\":{\"size\":[0,0],\"src\":\"default\",\"srcOrientation\":\"Right\"},\"iconOffset\":0,\"iconPlacement\":\"left\",\"opacity\":1,\"show\":true,\"text\":{\"content\":\"Reset Inputs\",\"font\":\"Arial\"}},\"labelOffset\":[0,0],\"verticalAlignment\":\"middle\"},{\"horizontalAlignment\":\"center\",\"image\":{\"position\":[0,0,1,1],\"size\":[1,1],\"src\":\"default\",\"srcOrientation\":\"Right\"},\"label\":{\"color\":[0.01176470588,0.01176470588,0.01176470588,1],\"icon\":{\"size\":[0,0],\"src\":\"default\",\"srcOrientation\":\"Right\"},\"iconOffset\":0,\"iconPlacement\":\"left\",\"opacity\":1,\"show\":true,\"text\":{\"content\":\"Reset Inputs\",\"font\":\"Arial\"}},\"labelOffset\":[0,0],\"verticalAlignment\":\"middle\"},{\"horizontalAlignment\":\"center\",\"image\":{\"position\":[0,0,1,1],\"size\":[1,1],\"src\":\"default\",\"srcOrientation\":\"Right\"},\"label\":{\"color\":[0.01176470588,0.01176470588,0.01176470588,1],\"icon\":{\"size\":[0,0],\"src\":\"default\",\"srcOrientation\":\"Right\"},\"iconOffset\":0,\"iconPlacement\":\"left\",\"opacity\":1,\"show\":true,\"text\":{\"content\":\"Reset Inputs\",\"font\":\"Arial\"}},\"labelOffset\":[0,0],\"verticalAlignment\":\"middle\"},{\"horizontalAlignment\":\"center\",\"image\":{\"position\":[0,0,1,1],\"size\":[1,1],\"src\":\"default\",\"srcOrientation\":\"Right\"},\"label\":{\"color\":[0.01176470588,0.01176470588,0.01176470588,1],\"icon\":{\"size\":[0,0],\"src\":\"default\",\"srcOrientation\":\"Right\"},\"iconOffset\":0,\"iconPlacement\":\"left\",\"opacity\":1,\"show\":true,\"text\":{\"content\":\"Reset Inputs\",\"font\":\"Arial\"}},\"labelOffset\":[0,0],\"verticalAlignment\":\"middle\"}]}},{\"name\":\"ForegroundImageComponent\",\"settings\":{\"image\":{\"size\":[0,0],\"src\":\"default\",\"srcOrientation\":\"Right\"},\"isForeground\":1,\"position\":[0,0,1,1]}}],\"settings\":{\"BindingType\":\"standalone\",\"backgroundColor\":[244,244,244,1],\"backgroundOffset\":0.2,\"backgroundOpacity\":1,\"fixedAspectRatio\":\"off\",\"foregroundColor\":[0.01176470588,0.01176470588,0.01176470588,1],\"migratedFromLegacy\":true,\"useBackgroundColor\":true,\"variant\":\"callback\",\"version\":\"R2023a\"},\"type\":\"Button\"}"  CustomBackgroundColor="{\"color\":[0.9568627451,0.9568627451,0.9568627451],\"show\":true}"
  Circle Pos : Constant  Value=-59.71488087488608
  Circle Shift : Constant  Value=0.1
  Constant : Constant  SampleTime=0.05
  Dashboard Input : sm_motor_grader_lib/Dashboard Input  upper_bound=motGradParams.articulation.upperBound  lower_bound=motGradParams.articulation.lowerBound  U0=motGradParams.articulation.initPos  tfilt=1
  Dashboard Input1 : sm_motor_grader_lib/Dashboard Input  upper_bound=motGradParams.circleRot.maxPos  lower_bound=motGradParams.circleRot.minPos  U0=motGradParams.circleRot.initPos  tfilt=0.1
  Dashboard Input2 : sm_motor_grader_lib/Dashboard Input  upper_bound=motGradParams.steer.upperBound  lower_bound=motGradParams.steer.lowerBound  U0=motGradParams.steer.initPos  tfilt=1
  Dashboard Input3 : sm_motor_grader_lib/Dashboard Input  upper_bound=motGradParams.wheelLean.upperBound  lower_bound=motGradParams.wheelLean.lowerBound  U0=motGradParams.wheelLean.initPos  tfilt=1
  Dashboard Input4 : sm_motor_grader_lib/Dashboard Input  upper_bound=motGradParams.bladeTilt.stroke  lower_bound=0  U0=motGradParams.bladeTilt.initPos  tfilt=0.1
  Dashboard Input5 : sm_motor_grader_lib/Dashboard Input  upper_bound=motGradParams.bladeLift.stroke  lower_bound=0  U0=motGradParams.bladeLift.leftInitPos  tfilt=0.1
  Dashboard Input6 : sm_motor_grader_lib/Dashboard Input  upper_bound=motGradParams.bladeLift.stroke  lower_bound=0  U0=motGradParams.bladeLift.rightInitPos  tfilt=0.1
  Dashboard Input7 : sm_motor_grader_lib/Dashboard Input  upper_bound=motGradParams.circleShift.stroke  lower_bound=0  U0=motGradParams.circleShift.initPos  tfilt=0.1
  Dashboard Input8 : sm_motor_grader_lib/Dashboard Input  upper_bound=motGradParams.bladeSideShift.stroke  lower_bound=0  U0=motGradParams.bladeSideShift.initPos  tfilt=0.1
  Dashboard Input9 : sm_motor_grader_lib/Dashboard Input  upper_bound=motGradParams.drivetrain.topSpeed  lower_bound=-motGradParams.drivetrain.topSpeed  U0=0  tfilt=1
  Lean : Constant  Value=0.166
  Lift L : Constant  Value=0.2666319489649785
  Lift R : Constant  Value=0.129983075120427
  Pin : Constant  Value=0
  Slider Blade Shift : SliderBlock  ScaleMax=1.3
  Slider Blade Tilt : SliderBlock  ScaleMax=0.20000000000000001
  Slider Circle Pos : SliderBlock  ScaleMin=-90  ScaleMax=90
  Slider Circle Shift : SliderBlock  ScaleMax=0.84999999999999998
  Slider Lift L : SliderBlock  ScaleMax=1.2
  Slider Lift R : SliderBlock  ScaleMax=1.2
  Steer : Constant  Value=0.20749
  Terminator : Terminator
  Terminator1 : Terminator
  Vehicle Speed : Constant  Value=0
  nHoleLink : Constant  Value=0
  nHoleLink1 : Constant  Value=0
  nHoleLink2 : Constant  Value=0
  Out Bus Element : Outport  PortName=Test  Element=pLean
  Out Bus Element1 : Outport  PortName=Test  Element=pSteer
  Out Bus Element2 : Outport  PortName=Test  Element=pArtic
  Out Bus Element5 : Outport  PortName=Test  Element=pLiftL
  Out Bus Element6 : Outport  PortName=Test  Element=pLiftR
  Out Bus Element7 : Outport  PortName=Test  Element=pCircleShift
  Out Bus Element8 : Outport  PortName=Test  Element=qCircle
  Out Bus Element9 : Outport  PortName=Test  Element=pTilt
  Out Bus Element10 : Outport  PortName=Test  Element=pShift
  Out Bus Element11 : Outport  PortName=Test  Element=vVeh
  Out Bus Element12 : Outport  PortName=Test  Element=nHoleLink
  Out Bus Element14 : Outport  PortName=Test  Element=pPin
  Out Bus Element13 : Outport  PortName=Test  Element=mLiftL
  Out Bus Element15 : Outport  PortName=Test  Element=mLiftR
  wires:
  Dashboard Input9/1 -> Out Bus Element11/1
  Vehicle Speed/1 -> Dashboard Input9/1
  Lift L/1 -> Dashboard Input5/1
  Lift R/1 -> Dashboard Input6/1
  Circle Shift/1 -> Dashboard Input7/1
  Circle Pos/1 -> Dashboard Input1/1
  Blade Tilt/1 -> Dashboard Input4/1
  Blade Shift/1 -> Dashboard Input8/1
  Lean/1 -> Dashboard Input3/1
  Steer/1 -> Dashboard Input2/1
  Dashboard Input/1 -> Out Bus Element2/1
  nHoleLink/1 -> Out Bus Element12/1
  Pin/1 -> Out Bus Element14/1
  Articulation/1 -> Dashboard Input/1
  Dashboard Input1/1 -> Out Bus Element8/1
  Dashboard Input2/1 -> Out Bus Element1/1
  Dashboard Input3/1 -> Out Bus Element/1
  Dashboard Input4/1 -> Out Bus Element9/1
  Dashboard Input5/1 -> Out Bus Element5/1
  Dashboard Input6/1 -> Out Bus Element6/1
  Dashboard Input7/1 -> Out Bus Element7/1
  Dashboard Input8/1 -> Out Bus Element10/1
  m/1 -> Terminator/1
  nHoleLink1/1 -> Out Bus Element13/1
  nHoleLink2/1 -> Out Bus Element15/1
  Constant/1 -> Terminator1/1

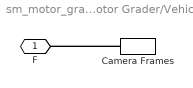
== system sm_motor_grader_LiftAssembly/Motor Grader/Vehicle ==
  Camera Frames : sm_vehicle_utilities_lib/Camera Frames  Camera=Camera  popup_dolly_camera=Off
  F : PMIOPort  Side=Right
  connections:
  Camera Frames/RConn1 -- F/RConn1
